simulink model "CVS Model"  (R2021a)
settings: Solver=VariableStepAuto  StartTime=0.0  StopTime=1.6  RelTol=1e-3
libraries: ee_lib x814, fl_lib x488, nesl_utility x60, simulink x4
(part 7 of 8)

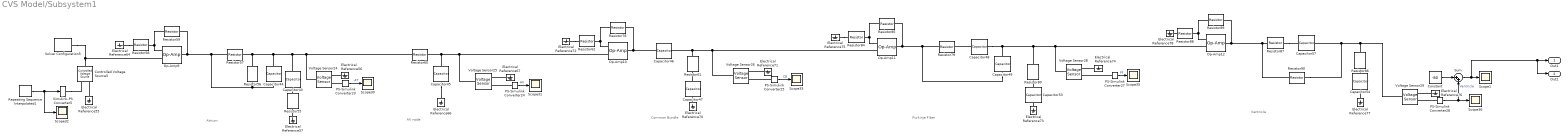
== system CVS Model/Subsystem1 ==
  note: Common Bundle
  note: Ventricle
  note: AV node
  note: Purkinje Fiber
  note: Atrium
  Capacitor43 : fl_lib/Electrical/Electrical Elements/Capacitor  c=80 uF  r=0 Ohm  g=0 1/Ohm  i_specify=off  i_priority=None  i=0 A  i_nominal_specify=off  i_nominal_unit=A  i_nominal_value=1  v_specify=off  v_priority=None  v=0 V  v_nominal_specify=off  v_nominal_unit=V  v_nominal_value=1  vc_specify=off  vc_priority=High  vc=0 V  vc_nominal_specify=off  vc_nominal_unit=V  vc_nominal_value=1
  Capacitor44 : fl_lib/Electrical/Electrical Elements/Capacitor  c=80 uF  r=0 Ohm  g=0 1/Ohm  i_specify=off  i_priority=None  i=0 A  i_nominal_specify=off  i_nominal_unit=A  i_nominal_value=1  v_specify=off  v_priority=None  v=0 V  v_nominal_specify=off  v_nominal_unit=V  v_nominal_value=1  vc_specify=off  vc_priority=High  vc=0 V  vc_nominal_specify=off  vc_nominal_unit=V  vc_nominal_value=1
  Capacitor45 : fl_lib/Electrical/Electrical Elements/Capacitor  c=20 uF  r=0 Ohm  g=0 1/Ohm  i_specify=off  i_priority=None  i=0 A  i_nominal_specify=off  i_nominal_unit=A  i_nominal_value=1  v_specify=off  v_priority=None  v=0 V  v_nominal_specify=off  v_nominal_unit=V  v_nominal_value=1  vc_specify=off  vc_priority=High  vc=0 V  vc_nominal_specify=off  vc_nominal_unit=V  vc_nominal_value=1
  Capacitor46 : fl_lib/Electrical/Electrical Elements/Capacitor  c=10 uF  r=1e-6 Ohm  g=0 1/Ohm  i_specify=off  i_priority=None  i=0 A  i_nominal_specify=off  i_nominal_unit=A  i_nominal_value=1  v_specify=off  v_priority=None  v=0 V  v_nominal_specify=off  v_nominal_unit=V  v_nominal_value=1  vc_specify=off  vc_priority=High  vc=0 V  vc_nominal_specify=off  vc_nominal_unit=V  vc_nominal_value=1
  Capacitor47 : fl_lib/Electrical/Electrical Elements/Capacitor  c=12 uF  r=0 Ohm  g=0 1/Ohm  i_specify=off  i_priority=None  i=0 A  i_nominal_specify=off  i_nominal_unit=A  i_nominal_value=1  v_specify=off  v_priority=None  v=0 V  v_nominal_specify=off  v_nominal_unit=V  v_nominal_value=1  vc_specify=off  vc_priority=High  vc=0 V  vc_nominal_specify=off  vc_nominal_unit=V  vc_nominal_value=1
  Capacitor48 : fl_lib/Electrical/Electrical Elements/Capacitor  c=20 uF  r=1e-6 Ohm  g=0 1/Ohm  i_specify=off  i_priority=None  i=0 A  i_nominal_specify=off  i_nominal_unit=A  i_nominal_value=1  v_specify=off  v_priority=None  v=0 V  v_nominal_specify=off  v_nominal_unit=V  v_nominal_value=1  vc_specify=off  vc_priority=High  vc=0 V  vc_nominal_specify=off  vc_nominal_unit=V  vc_nominal_value=1
  Capacitor49 : fl_lib/Electrical/Electrical Elements/Capacitor  c=30 uF  r=1e-6 Ohm  g=0 1/Ohm  i_specify=off  i_priority=None  i=0 A  i_nominal_specify=off  i_nominal_unit=A  i_nominal_value=1  v_specify=off  v_priority=None  v=0 V  v_nominal_specify=off  v_nominal_unit=V  v_nominal_value=1  vc_specify=off  vc_priority=High  vc=0 V  vc_nominal_specify=off  vc_nominal_unit=V  vc_nominal_value=1
  Capacitor53 : fl_lib/Electrical/Electrical Elements/Capacitor  c=50 uF  r=1e-6 Ohm  g=0 1/Ohm  i_specify=off  i_priority=None  i=0 A  i_nominal_specify=off  i_nominal_unit=A  i_nominal_value=1  v_specify=off  v_priority=None  v=0 V  v_nominal_specify=off  v_nominal_unit=V  v_nominal_value=1  vc_specify=off  vc_priority=High  vc=0 V  vc_nominal_specify=off  vc_nominal_unit=V  vc_nominal_value=1
  Capacitor54 : fl_lib/Electrical/Electrical Elements/Capacitor  c=2.5 uF  r=0 Ohm  g=0 1/Ohm  i_specify=off  i_priority=None  i=0 A  i_nominal_specify=off  i_nominal_unit=A  i_nominal_value=1  v_specify=off  v_priority=None  v=0 V  v_nominal_specify=off  v_nominal_unit=V  v_nominal_value=1  vc_specify=off  vc_priority=High  vc=0 V  vc_nominal_specify=off  vc_nominal_unit=V  vc_nominal_value=1
  Capacitor57 : fl_lib/Electrical/Electrical Elements/Capacitor  c=8 uF  r=0 Ohm  g=0 1/Ohm  i_specify=off  i_priority=None  i=0 A  i_nominal_specify=off  i_nominal_unit=A  i_nominal_value=1  v_specify=off  v_priority=None  v=0 V  v_nominal_specify=off  v_nominal_unit=V  v_nominal_value=1  vc_specify=off  vc_priority=High  vc=0 V  vc_nominal_specify=off  vc_nominal_unit=V  vc_nominal_value=1
  Constant : Constant  Value=-80
  Controlled Voltage Source5 : fl_lib/Electrical/Electrical Sources/Controlled Voltage Source
  Electrical Reference{55..57,64,66..67,70..78} (15 alike) : fl_lib/Electrical/Electrical Elements/Electrical Reference
  Op-Amp{9..12} (4 alike) : fl_lib/Electrical/Electrical Elements/Op-Amp  outI_specify=off  outI_priority=None  outI=0 A  outI_nominal_specify=off  outI_nominal_unit=A  outI_nominal_value=1
  PS-Simulink Converter{23..25,27..28} (5 alike) : nesl_utility/PS-Simulink Converter  PhysicalDomain=network_engine_domain  SubClassName=ps_output  LeftPortType=input  RightPortType=output  PseudoPeriodic=off  Frequencies=[]  Unit=inherit  AffineConversion=off
      settings: SourceProductBaseCode=PW,SS
  Repeating Sequence Interpolated1 : simulink/Sources/Repeating Sequence Interpolated  OutValues=[0 0.01 60 -3 0].'  TimeValues=[0 0.1 0.12 0.4 0.8].'  LookUpMeth=Interpolation-Use End Values  tsamp=0.0001  OutMin=[]  OutMax=[]  OutDataTypeStr=double  OutputDataTypeScalingMode=double  OutDataType=fixdt(0,8)  OutScaling=2^-10
  Resistor55 : fl_lib/Electrical/Electrical Elements/Resistor  R=0.4 kOhm  i_specify=off  i_priority=None  i=0 A  i_nominal_specify=off  i_nominal_unit=A  i_nominal_value=1  v_specify=off  v_priority=None  v=0 V  v_nominal_specify=off  v_nominal_unit=V  v_nominal_value=1
  Resistor56 : fl_lib/Electrical/Electrical Elements/Resistor  R=40 kOhm  i_specify=off  i_priority=None  i=0 A  i_nominal_specify=off  i_nominal_unit=A  i_nominal_value=1  v_specify=off  v_priority=None  v=0 V  v_nominal_specify=off  v_nominal_unit=V  v_nominal_value=1
  Resistor57 : fl_lib/Electrical/Electrical Elements/Resistor  R=0.3 kOhm  i_specify=off  i_priority=None  i=0 A  i_nominal_specify=off  i_nominal_unit=A  i_nominal_value=1  v_specify=off  v_priority=None  v=0 V  v_nominal_specify=off  v_nominal_unit=V  v_nominal_value=1
  Resistor58 : fl_lib/Electrical/Electrical Elements/Resistor  R=2 kOhm  i_specify=off  i_priority=None  i=0 A  i_nominal_specify=off  i_nominal_unit=A  i_nominal_value=1  v_specify=off  v_priority=None  v=0 V  v_nominal_specify=off  v_nominal_unit=V  v_nominal_value=1
  Resistor{59,78,85,89} (4 alike) : fl_lib/Electrical/Electrical Elements/Resistor  R=1.5 kOhm  i_specify=off  i_priority=None  i=0 A  i_nominal_specify=off  i_nominal_unit=A  i_nominal_value=1  v_specify=off  v_priority=None  v=0 V  v_nominal_specify=off  v_nominal_unit=V  v_nominal_value=1
  Resistor60 : fl_lib/Electrical/Electrical Elements/Resistor  R=0.4 kOhm  i_specify=off  i_priority=None  i=0 A  i_nominal_specify=off  i_nominal_unit=A  i_nominal_value=1  v_specify=off  v_priority=None  v=0 V  v_nominal_specify=off  v_nominal_unit=V  v_nominal_value=1
  Resistor61 : fl_lib/Electrical/Electrical Elements/Resistor  R=0.5 kOhm  i_specify=off  i_priority=None  i=0 A  i_nominal_specify=off  i_nominal_unit=A  i_nominal_value=1  v_specify=off  v_priority=None  v=0 V  v_nominal_specify=off  v_nominal_unit=V  v_nominal_value=1
  Resistor62 : fl_lib/Electrical/Electrical Elements/Resistor  R=2 kOhm  i_specify=off  i_priority=None  i=0 A  i_nominal_specify=off  i_nominal_unit=A  i_nominal_value=1  v_specify=off  v_priority=None  v=0 V  v_nominal_specify=off  v_nominal_unit=V  v_nominal_value=1
  Resistor79 : fl_lib/Electrical/Electrical Elements/Resistor  R=0.2 kOhm  i_specify=off  i_priority=None  i=0 A  i_nominal_specify=off  i_nominal_unit=A  i_nominal_value=1  v_specify=off  v_priority=None  v=0 V  v_nominal_specify=off  v_nominal_unit=V  v_nominal_value=1
  Resistor80 : fl_lib/Electrical/Electrical Elements/Resistor  R=0.4 kOhm  i_specify=off  i_priority=None  i=0 A  i_nominal_specify=off  i_nominal_unit=A  i_nominal_value=1  v_specify=off  v_priority=None  v=0 V  v_nominal_specify=off  v_nominal_unit=V  v_nominal_value=1
  Resistor84 : fl_lib/Electrical/Electrical Elements/Resistor  R=0.7 kOhm  i_specify=off  i_priority=None  i=0 A  i_nominal_specify=off  i_nominal_unit=A  i_nominal_value=1  v_specify=off  v_priority=None  v=0 V  v_nominal_specify=off  v_nominal_unit=V  v_nominal_value=1
  Resistor86 : fl_lib/Electrical/Electrical Elements/Resistor  R=1 kOhm  i_specify=off  i_priority=None  i=0 A  i_nominal_specify=off  i_nominal_unit=A  i_nominal_value=1  v_specify=off  v_priority=None  v=0 V  v_nominal_specify=off  v_nominal_unit=V  v_nominal_value=1
  Resistor87 : fl_lib/Electrical/Electrical Elements/Resistor  R=0.5 kOhm  i_specify=off  i_priority=None  i=0 A  i_nominal_specify=off  i_nominal_unit=A  i_nominal_value=1  v_specify=off  v_priority=None  v=0 V  v_nominal_specify=off  v_nominal_unit=V  v_nominal_value=1
  Resistor88 : fl_lib/Electrical/Electrical Elements/Resistor  R=3.5 kOhm  i_specify=off  i_priority=None  i=0 A  i_nominal_specify=off  i_nominal_unit=A  i_nominal_value=1  v_specify=off  v_priority=None  v=0 V  v_nominal_specify=off  v_nominal_unit=V  v_nominal_value=1
  Resistor90 : fl_lib/Electrical/Electrical Elements/Resistor  R=2.5 kOhm  i_specify=off  i_priority=None  i=0 A  i_nominal_specify=off  i_nominal_unit=A  i_nominal_value=1  v_specify=off  v_priority=None  v=0 V  v_nominal_specify=off  v_nominal_unit=V  v_nominal_value=1
  Scope{1,30..33,35..36} (7 alike) : Scope
  Simulink-PS Converter5 : nesl_utility/Simulink-PS Converter  PhysicalDomain=network_engine_domain  SubClassName=ps_input  LeftPortType=input  RightPortType=output  PseudoPeriodic=off  Frequencies=[]  NoiseDistribution=none  NoiseParameters=[]  Unit=1  AffineConversion=off  FilteringAndDerivatives=provide  SimscapeFilterOrder=1  InputFilterTimeConstant=0.001  UdotUserProvided=0
      settings: SourceProductBaseCode=PW,SS
  Solver Configuration5 : nesl_utility/Solver Configuration  PhysicalDomain=network_engine_domain  SubClassName=solver  LeftPortType=input  RightPortType=generic  Tones=[]  Harmonics=[]  SimulateNoise=off  Profile=off  UseLocalSampling=off  EnableSwitchedLinearOptims=on  FrequencyDomain=off  UseCCode=off  RelTol=0.001  AbsTol=1e-06  MinStep=1e-09  ToWorkspace=off  RevertToSquareIcSolve=off  NumHomotopyIterations=100  PhasorMode=off  PhasorModeNumHarmonics=1  DoDC=off  ResidualTolerance=1e-09  UseLocalSolver=off  LocalSolverChoice=NE_BACKWARD_EULER_ADVANCER  LocalSolverSampleTime=0.001  DoFixedCost=off  MaxNonlinIter=3  MaxModeIter=2  ComputeImpulses=off  ImpulseIterations=2  LinearAlgebra=auto  EquationFormulation=NE_TIME_EF  DelaysMemoryBudget=1024  AutomaticFiltering=on  FilteringTimeConstant=0.001  PartitionStorageMethod=AS_NEEDED  PartitionMemoryBudget=1024  PartitionMethod=ROBUST
      settings: SourceProductBaseCode=PW,SS
  Sum : Sum  Inputs=|++
  Voltage Sensor{24..26,28..29} (5 alike) : fl_lib/Electrical/Electrical Sensors/Voltage Sensor
  Out1 : Outport
  Out2 : Outport  Port=2
  wires:
  Repeating Sequence Interpolated1/1 -> Scope32/1, Simulink-PS Converter5/1
  PS-Simulink Converter24/1 -> Scope31/1  "AV"
  PS-Simulink Converter28/1 -> Sum/2, Scope36/1  "Ventricle"
  PS-Simulink Converter25/1 -> Scope33/1  "CB"
  PS-Simulink Converter23/1 -> Scope30/1  "AT"
  PS-Simulink Converter27/1 -> Scope35/1  "PF"
  Sum/1 -> Out2/1, Out1/1, Scope1/1
  Constant/1 -> Sum/1
  connections:
  PS-Simulink Converter24/LConn1 -- Voltage Sensor25/RConn1
  Resistor86/RConn1 -- Capacitor54/LConn1
  Resistor56/RConn1 -- Capacitor44/RConn1 -- Resistor57/LConn1 -- Resistor59/RConn1 -- Op-Amp9/RConn1
  Capacitor45/LConn1 -- Resistor60/RConn1 -- Op-Amp10/LConn2 -- Voltage Sensor25/LConn1
  Capacitor46/LConn1 -- Resistor78/RConn1 -- Op-Amp10/RConn1
  Electrical Reference55/LConn1 -- Controlled Voltage Source5/RConn2
  PS-Simulink Converter27/LConn1 -- Voltage Sensor28/RConn1
  Electrical Reference76/LConn1 -- Voltage Sensor29/RConn2
  Resistor85/RConn1 -- Op-Amp11/RConn1 -- Resistor79/LConn1 -- Capacitor49/RConn1
  Resistor89/RConn1 -- Op-Amp12/RConn1 -- Resistor87/LConn1 -- Resistor90/RConn1
  Electrical Reference78/LConn1 -- Resistor88/LConn1
  Resistor84/RConn1 -- Resistor85/LConn1 -- Op-Amp11/LConn1
  Resistor90/LConn1 -- Voltage Sensor29/LConn1 -- Resistor86/LConn1 -- Capacitor57/RConn1
  PS-Simulink Converter23/LConn1 -- Voltage Sensor24/RConn1
  Capacitor53/RConn1 -- Electrical Reference73/LConn1
  Capacitor47/RConn1 -- Electrical Reference70/LConn1
  Capacitor53/LConn1 -- Resistor80/RConn1
  PS-Simulink Converter28/LConn1 -- Voltage Sensor29/RConn1
  Controlled Voltage Source5/LConn1 -- Solver Configuration5/RConn1 -- Op-Amp9/LConn2
  Resistor62/RConn1 -- Resistor78/LConn1 -- Op-Amp10/LConn1
  Electrical Reference72/LConn1 -- Resistor62/LConn1
  Simulink-PS Converter5/RConn1 -- Controlled Voltage Source5/RConn1
  Electrical Reference64/LConn1 -- Resistor58/LConn1
  Capacitor45/RConn1 -- Electrical Reference66/LConn1
  PS-Simulink Converter25/LConn1 -- Voltage Sensor26/RConn1
  Electrical Reference75/LConn1 -- Resistor84/LConn1
  Capacitor48/LConn1 -- Resistor79/RConn1
  Electrical Reference74/LConn1 -- Voltage Sensor28/RConn2
  Electrical Reference71/LConn1 -- Voltage Sensor26/RConn2
  Resistor87/RConn1 -- Capacitor57/LConn1
  Electrical Reference67/LConn1 -- Voltage Sensor25/RConn2
  Electrical Reference77/LConn1 -- Capacitor54/RConn1
  Capacitor47/LConn1 -- Resistor61/RConn1
  Electrical Reference57/LConn1 -- Resistor55/RConn1
  Electrical Reference56/LConn1 -- Voltage Sensor24/RConn2
  Capacitor43/RConn1 -- Resistor55/LConn1
  Capacitor43/LConn1 -- Capacitor44/LConn1 -- Resistor56/LConn1 -- Resistor57/RConn1 -- Resistor60/LConn1 -- Voltage Sensor24/LConn1
  Resistor88/RConn1 -- Op-Amp12/LConn1 -- Resistor89/LConn1
  Resistor58/RConn1 -- Op-Amp9/LConn1 -- Resistor59/LConn1
  Voltage Sensor28/LConn1 -- Op-Amp12/LConn2 -- Resistor80/LConn1 -- Capacitor48/RConn1 -- Capacitor49/LConn1
  Capacitor46/RConn1 -- Resistor61/LConn1 -- Op-Amp11/LConn2 -- Voltage Sensor26/LConn1

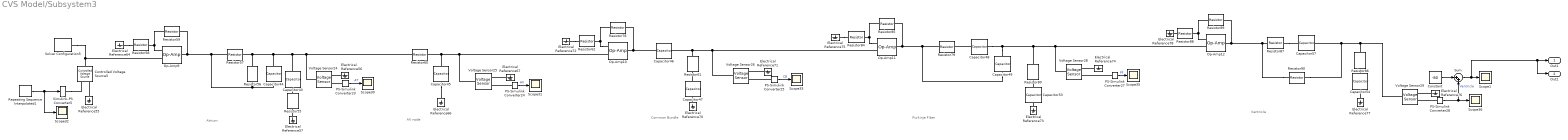
== system CVS Model/Subsystem3 ==
  note: Atrium
  note: Purkinje Fiber
  note: AV node
  note: Ventricle
  note: Common Bundle
  Capacitor43 : fl_lib/Electrical/Electrical Elements/Capacitor  c=80 uF  r=0 Ohm  g=0 1/Ohm  i_specify=off  i_priority=None  i=0 A  i_nominal_specify=off  i_nominal_unit=A  i_nominal_value=1  v_specify=off  v_priority=None  v=0 V  v_nominal_specify=off  v_nominal_unit=V  v_nominal_value=1  vc_specify=off  vc_priority=High  vc=0 V  vc_nominal_specify=off  vc_nominal_unit=V  vc_nominal_value=1
  Capacitor44 : fl_lib/Electrical/Electrical Elements/Capacitor  c=80 uF  r=0 Ohm  g=0 1/Ohm  i_specify=off  i_priority=None  i=0 A  i_nominal_specify=off  i_nominal_unit=A  i_nominal_value=1  v_specify=off  v_priority=None  v=0 V  v_nominal_specify=off  v_nominal_unit=V  v_nominal_value=1  vc_specify=off  vc_priority=High  vc=0 V  vc_nominal_specify=off  vc_nominal_unit=V  vc_nominal_value=1
  Capacitor45 : fl_lib/Electrical/Electrical Elements/Capacitor  c=20 uF  r=0 Ohm  g=0 1/Ohm  i_specify=off  i_priority=None  i=0 A  i_nominal_specify=off  i_nominal_unit=A  i_nominal_value=1  v_specify=off  v_priority=None  v=0 V  v_nominal_specify=off  v_nominal_unit=V  v_nominal_value=1  vc_specify=off  vc_priority=High  vc=0 V  vc_nominal_specify=off  vc_nominal_unit=V  vc_nominal_value=1
  Capacitor46 : fl_lib/Electrical/Electrical Elements/Capacitor  c=10 uF  r=1e-6 Ohm  g=0 1/Ohm  i_specify=off  i_priority=None  i=0 A  i_nominal_specify=off  i_nominal_unit=A  i_nominal_value=1  v_specify=off  v_priority=None  v=0 V  v_nominal_specify=off  v_nominal_unit=V  v_nominal_value=1  vc_specify=off  vc_priority=High  vc=0 V  vc_nominal_specify=off  vc_nominal_unit=V  vc_nominal_value=1
  Capacitor47 : fl_lib/Electrical/Electrical Elements/Capacitor  c=12 uF  r=0 Ohm  g=0 1/Ohm  i_specify=off  i_priority=None  i=0 A  i_nominal_specify=off  i_nominal_unit=A  i_nominal_value=1  v_specify=off  v_priority=None  v=0 V  v_nominal_specify=off  v_nominal_unit=V  v_nominal_value=1  vc_specify=off  vc_priority=High  vc=0 V  vc_nominal_specify=off  vc_nominal_unit=V  vc_nominal_value=1
  Capacitor48 : fl_lib/Electrical/Electrical Elements/Capacitor  c=20 uF  r=1e-6 Ohm  g=0 1/Ohm  i_specify=off  i_priority=None  i=0 A  i_nominal_specify=off  i_nominal_unit=A  i_nominal_value=1  v_specify=off  v_priority=None  v=0 V  v_nominal_specify=off  v_nominal_unit=V  v_nominal_value=1  vc_specify=off  vc_priority=High  vc=0 V  vc_nominal_specify=off  vc_nominal_unit=V  vc_nominal_value=1
  Capacitor49 : fl_lib/Electrical/Electrical Elements/Capacitor  c=30 uF  r=1e-6 Ohm  g=0 1/Ohm  i_specify=off  i_priority=None  i=0 A  i_nominal_specify=off  i_nominal_unit=A  i_nominal_value=1  v_specify=off  v_priority=None  v=0 V  v_nominal_specify=off  v_nominal_unit=V  v_nominal_value=1  vc_specify=off  vc_priority=High  vc=0 V  vc_nominal_specify=off  vc_nominal_unit=V  vc_nominal_value=1
  Capacitor53 : fl_lib/Electrical/Electrical Elements/Capacitor  c=50 uF  r=1e-6 Ohm  g=0 1/Ohm  i_specify=off  i_priority=None  i=0 A  i_nominal_specify=off  i_nominal_unit=A  i_nominal_value=1  v_specify=off  v_priority=None  v=0 V  v_nominal_specify=off  v_nominal_unit=V  v_nominal_value=1  vc_specify=off  vc_priority=High  vc=0 V  vc_nominal_specify=off  vc_nominal_unit=V  vc_nominal_value=1
  Capacitor54 : fl_lib/Electrical/Electrical Elements/Capacitor  c=2.5 uF  r=0 Ohm  g=0 1/Ohm  i_specify=off  i_priority=None  i=0 A  i_nominal_specify=off  i_nominal_unit=A  i_nominal_value=1  v_specify=off  v_priority=None  v=0 V  v_nominal_specify=off  v_nominal_unit=V  v_nominal_value=1  vc_specify=off  vc_priority=High  vc=0 V  vc_nominal_specify=off  vc_nominal_unit=V  vc_nominal_value=1
  Capacitor57 : fl_lib/Electrical/Electrical Elements/Capacitor  c=8 uF  r=0 Ohm  g=0 1/Ohm  i_specify=off  i_priority=None  i=0 A  i_nominal_specify=off  i_nominal_unit=A  i_nominal_value=1  v_specify=off  v_priority=None  v=0 V  v_nominal_specify=off  v_nominal_unit=V  v_nominal_value=1  vc_specify=off  vc_priority=High  vc=0 V  vc_nominal_specify=off  vc_nominal_unit=V  vc_nominal_value=1
  Constant : Constant  Value=-80
  Controlled Voltage Source5 : fl_lib/Electrical/Electrical Sources/Controlled Voltage Source
  Electrical Reference{55..57,64,66..67,70..78} (15 alike) : fl_lib/Electrical/Electrical Elements/Electrical Reference
  Op-Amp{9..12} (4 alike) : fl_lib/Electrical/Electrical Elements/Op-Amp  outI_specify=off  outI_priority=None  outI=0 A  outI_nominal_specify=off  outI_nominal_unit=A  outI_nominal_value=1
  PS-Simulink Converter{23..25,27..28} (5 alike) : nesl_utility/PS-Simulink Converter  PhysicalDomain=network_engine_domain  SubClassName=ps_output  LeftPortType=input  RightPortType=output  PseudoPeriodic=off  Frequencies=[]  Unit=inherit  AffineConversion=off
      settings: SourceProductBaseCode=PW,SS
  Repeating Sequence Interpolated1 : simulink/Sources/Repeating Sequence Interpolated  OutValues=[0 0.01 60 -3 0].'  TimeValues=[0 0.1 0.12 0.4 0.8].'  LookUpMeth=Interpolation-Use End Values  tsamp=0.0001  OutMin=[]  OutMax=[]  OutDataTypeStr=double  OutputDataTypeScalingMode=double  OutDataType=fixdt(0,8)  OutScaling=2^-10
  Resistor55 : fl_lib/Electrical/Electrical Elements/Resistor  R=0.4 kOhm  i_specify=off  i_priority=None  i=0 A  i_nominal_specify=off  i_nominal_unit=A  i_nominal_value=1  v_specify=off  v_priority=None  v=0 V  v_nominal_specify=off  v_nominal_unit=V  v_nominal_value=1
  Resistor56 : fl_lib/Electrical/Electrical Elements/Resistor  R=40 kOhm  i_specify=off  i_priority=None  i=0 A  i_nominal_specify=off  i_nominal_unit=A  i_nominal_value=1  v_specify=off  v_priority=None  v=0 V  v_nominal_specify=off  v_nominal_unit=V  v_nominal_value=1
  Resistor57 : fl_lib/Electrical/Electrical Elements/Resistor  R=0.3 kOhm  i_specify=off  i_priority=None  i=0 A  i_nominal_specify=off  i_nominal_unit=A  i_nominal_value=1  v_specify=off  v_priority=None  v=0 V  v_nominal_specify=off  v_nominal_unit=V  v_nominal_value=1
  Resistor58 : fl_lib/Electrical/Electrical Elements/Resistor  R=2 kOhm  i_specify=off  i_priority=None  i=0 A  i_nominal_specify=off  i_nominal_unit=A  i_nominal_value=1  v_specify=off  v_priority=None  v=0 V  v_nominal_specify=off  v_nominal_unit=V  v_nominal_value=1
  Resistor{59,78,85,89} (4 alike) : fl_lib/Electrical/Electrical Elements/Resistor  R=1.5 kOhm  i_specify=off  i_priority=None  i=0 A  i_nominal_specify=off  i_nominal_unit=A  i_nominal_value=1  v_specify=off  v_priority=None  v=0 V  v_nominal_specify=off  v_nominal_unit=V  v_nominal_value=1
  Resistor60 : fl_lib/Electrical/Electrical Elements/Resistor  R=0.4 kOhm  i_specify=off  i_priority=None  i=0 A  i_nominal_specify=off  i_nominal_unit=A  i_nominal_value=1  v_specify=off  v_priority=None  v=0 V  v_nominal_specify=off  v_nominal_unit=V  v_nominal_value=1
  Resistor61 : fl_lib/Electrical/Electrical Elements/Resistor  R=0.5 kOhm  i_specify=off  i_priority=None  i=0 A  i_nominal_specify=off  i_nominal_unit=A  i_nominal_value=1  v_specify=off  v_priority=None  v=0 V  v_nominal_specify=off  v_nominal_unit=V  v_nominal_value=1
  Resistor62 : fl_lib/Electrical/Electrical Elements/Resistor  R=2 kOhm  i_specify=off  i_priority=None  i=0 A  i_nominal_specify=off  i_nominal_unit=A  i_nominal_value=1  v_specify=off  v_priority=None  v=0 V  v_nominal_specify=off  v_nominal_unit=V  v_nominal_value=1
  Resistor79 : fl_lib/Electrical/Electrical Elements/Resistor  R=0.2 kOhm  i_specify=off  i_priority=None  i=0 A  i_nominal_specify=off  i_nominal_unit=A  i_nominal_value=1  v_specify=off  v_priority=None  v=0 V  v_nominal_specify=off  v_nominal_unit=V  v_nominal_value=1
  Resistor80 : fl_lib/Electrical/Electrical Elements/Resistor  R=0.4 kOhm  i_specify=off  i_priority=None  i=0 A  i_nominal_specify=off  i_nominal_unit=A  i_nominal_value=1  v_specify=off  v_priority=None  v=0 V  v_nominal_specify=off  v_nominal_unit=V  v_nominal_value=1
  Resistor84 : fl_lib/Electrical/Electrical Elements/Resistor  R=0.7 kOhm  i_specify=off  i_priority=None  i=0 A  i_nominal_specify=off  i_nominal_unit=A  i_nominal_value=1  v_specify=off  v_priority=None  v=0 V  v_nominal_specify=off  v_nominal_unit=V  v_nominal_value=1
  Resistor86 : fl_lib/Electrical/Electrical Elements/Resistor  R=1 kOhm  i_specify=off  i_priority=None  i=0 A  i_nominal_specify=off  i_nominal_unit=A  i_nominal_value=1  v_specify=off  v_priority=None  v=0 V  v_nominal_specify=off  v_nominal_unit=V  v_nominal_value=1
  Resistor87 : fl_lib/Electrical/Electrical Elements/Resistor  R=5 kOhm  i_specify=off  i_priority=None  i=0 A  i_nominal_specify=off  i_nominal_unit=A  i_nominal_value=1  v_specify=off  v_priority=None  v=0 V  v_nominal_specify=off  v_nominal_unit=V  v_nominal_value=1
  Resistor88 : fl_lib/Electrical/Electrical Elements/Resistor  R=3.5 kOhm  i_specify=off  i_priority=None  i=0 A  i_nominal_specify=off  i_nominal_unit=A  i_nominal_value=1  v_specify=off  v_priority=None  v=0 V  v_nominal_specify=off  v_nominal_unit=V  v_nominal_value=1
  Resistor90 : fl_lib/Electrical/Electrical Elements/Resistor  R=2.5 kOhm  i_specify=off  i_priority=None  i=0 A  i_nominal_specify=off  i_nominal_unit=A  i_nominal_value=1  v_specify=off  v_priority=None  v=0 V  v_nominal_specify=off  v_nominal_unit=V  v_nominal_value=1
  Scope{1,30..33,35..36} (7 alike) : Scope
  Simulink-PS Converter5 : nesl_utility/Simulink-PS Converter  PhysicalDomain=network_engine_domain  SubClassName=ps_input  LeftPortType=input  RightPortType=output  PseudoPeriodic=off  Frequencies=[]  NoiseDistribution=none  NoiseParameters=[]  Unit=1  AffineConversion=off  FilteringAndDerivatives=provide  SimscapeFilterOrder=1  InputFilterTimeConstant=0.001  UdotUserProvided=0
      settings: SourceProductBaseCode=PW,SS
  Solver Configuration5 : nesl_utility/Solver Configuration  PhysicalDomain=network_engine_domain  SubClassName=solver  LeftPortType=input  RightPortType=generic  Tones=[]  Harmonics=[]  SimulateNoise=off  Profile=off  UseLocalSampling=off  EnableSwitchedLinearOptims=on  FrequencyDomain=off  UseCCode=off  RelTol=0.001  AbsTol=1e-06  MinStep=1e-09  ToWorkspace=off  RevertToSquareIcSolve=off  NumHomotopyIterations=100  PhasorMode=off  PhasorModeNumHarmonics=1  DoDC=off  ResidualTolerance=1e-09  UseLocalSolver=off  LocalSolverChoice=NE_BACKWARD_EULER_ADVANCER  LocalSolverSampleTime=0.001  DoFixedCost=off  MaxNonlinIter=3  MaxModeIter=2  ComputeImpulses=off  ImpulseIterations=2  LinearAlgebra=auto  EquationFormulation=NE_TIME_EF  DelaysMemoryBudget=1024  AutomaticFiltering=on  FilteringTimeConstant=0.001  PartitionStorageMethod=AS_NEEDED  PartitionMemoryBudget=1024  PartitionMethod=ROBUST
      settings: SourceProductBaseCode=PW,SS
  Sum : Sum  Inputs=|++
  Voltage Sensor{24..26,28..29} (5 alike) : fl_lib/Electrical/Electrical Sensors/Voltage Sensor
  Out1 : Outport
  Out2 : Outport  Port=2
  wires:
  Constant/1 -> Sum/1
  Sum/1 -> Scope1/1, Out1/1, Out2/1
  PS-Simulink Converter27/1 -> Scope35/1  "PF"
  PS-Simulink Converter23/1 -> Scope30/1  "AT"
  PS-Simulink Converter25/1 -> Scope33/1  "CB"
  PS-Simulink Converter28/1 -> Scope36/1, Sum/2  "Ventricle"
  PS-Simulink Converter24/1 -> Scope31/1  "AV"
  Repeating Sequence Interpolated1/1 -> Simulink-PS Converter5/1, Scope32/1
  connections:
  Voltage Sensor26/LConn1 -- Op-Amp11/LConn2 -- Resistor61/LConn1 -- Capacitor46/RConn1
  Capacitor49/LConn1 -- Capacitor48/RConn1 -- Resistor80/LConn1 -- Op-Amp12/LConn2 -- Voltage Sensor28/LConn1
  Resistor59/LConn1 -- Op-Amp9/LConn1 -- Resistor58/RConn1
  Resistor89/LConn1 -- Op-Amp12/LConn1 -- Resistor88/RConn1
  Voltage Sensor24/LConn1 -- Resistor60/LConn1 -- Resistor57/RConn1 -- Resistor56/LConn1 -- Capacitor44/LConn1 -- Capacitor43/LConn1
  Capacitor43/RConn1 -- Resistor55/LConn1
  Electrical Reference56/LConn1 -- Voltage Sensor24/RConn2
  Electrical Reference57/LConn1 -- Resistor55/RConn1
  Capacitor47/LConn1 -- Resistor61/RConn1
  Electrical Reference77/LConn1 -- Capacitor54/RConn1
  Electrical Reference67/LConn1 -- Voltage Sensor25/RConn2
  Resistor87/RConn1 -- Capacitor57/LConn1
  Electrical Reference71/LConn1 -- Voltage Sensor26/RConn2
  Electrical Reference74/LConn1 -- Voltage Sensor28/RConn2
  Capacitor48/LConn1 -- Resistor79/RConn1
  Electrical Reference75/LConn1 -- Resistor84/LConn1
  PS-Simulink Converter25/LConn1 -- Voltage Sensor26/RConn1
  Capacitor45/RConn1 -- Electrical Reference66/LConn1
  Electrical Reference64/LConn1 -- Resistor58/LConn1
  Simulink-PS Converter5/RConn1 -- Controlled Voltage Source5/RConn1
  Electrical Reference72/LConn1 -- Resistor62/LConn1
  Op-Amp10/LConn1 -- Resistor78/LConn1 -- Resistor62/RConn1
  Op-Amp9/LConn2 -- Solver Configuration5/RConn1 -- Controlled Voltage Source5/LConn1
  PS-Simulink Converter28/LConn1 -- Voltage Sensor29/RConn1
  Capacitor53/LConn1 -- Resistor80/RConn1
  Capacitor47/RConn1 -- Electrical Reference70/LConn1
  Capacitor53/RConn1 -- Electrical Reference73/LConn1
  PS-Simulink Converter23/LConn1 -- Voltage Sensor24/RConn1
  Capacitor57/RConn1 -- Resistor86/LConn1 -- Voltage Sensor29/LConn1 -- Resistor90/LConn1
  Op-Amp11/LConn1 -- Resistor85/LConn1 -- Resistor84/RConn1
  Electrical Reference78/LConn1 -- Resistor88/LConn1
  Resistor90/RConn1 -- Resistor87/LConn1 -- Op-Amp12/RConn1 -- Resistor89/RConn1
  Capacitor49/RConn1 -- Resistor79/LConn1 -- Op-Amp11/RConn1 -- Resistor85/RConn1
  Electrical Reference76/LConn1 -- Voltage Sensor29/RConn2
  PS-Simulink Converter27/LConn1 -- Voltage Sensor28/RConn1
  Electrical Reference55/LConn1 -- Controlled Voltage Source5/RConn2
  Op-Amp10/RConn1 -- Resistor78/RConn1 -- Capacitor46/LConn1
  Voltage Sensor25/LConn1 -- Op-Amp10/LConn2 -- Resistor60/RConn1 -- Capacitor45/LConn1
  Op-Amp9/RConn1 -- Resistor59/RConn1 -- Resistor57/LConn1 -- Capacitor44/RConn1 -- Resistor56/RConn1
  Resistor86/RConn1 -- Capacitor54/LConn1
  PS-Simulink Converter24/LConn1 -- Voltage Sensor25/RConn1

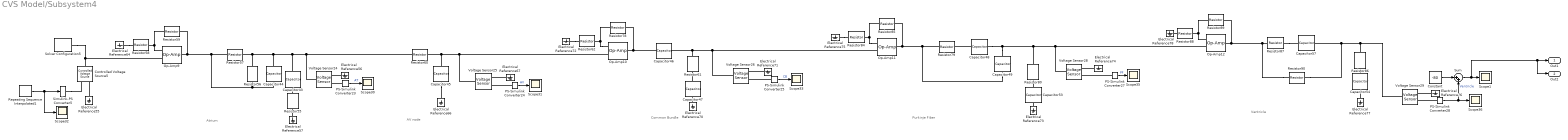
== system CVS Model/Subsystem4 ==
  note: Atrium
  note: Purkinje Fiber
  note: AV node
  note: Ventricle
  note: Common Bundle
  Capacitor43 : fl_lib/Electrical/Electrical Elements/Capacitor  c=80 uF  r=0 Ohm  g=0 1/Ohm  i_specify=off  i_priority=None  i=0 A  i_nominal_specify=off  i_nominal_unit=A  i_nominal_value=1  v_specify=off  v_priority=None  v=0 V  v_nominal_specify=off  v_nominal_unit=V  v_nominal_value=1  vc_specify=off  vc_priority=High  vc=0 V  vc_nominal_specify=off  vc_nominal_unit=V  vc_nominal_value=1
  Capacitor44 : fl_lib/Electrical/Electrical Elements/Capacitor  c=80 uF  r=0 Ohm  g=0 1/Ohm  i_specify=off  i_priority=None  i=0 A  i_nominal_specify=off  i_nominal_unit=A  i_nominal_value=1  v_specify=off  v_priority=None  v=0 V  v_nominal_specify=off  v_nominal_unit=V  v_nominal_value=1  vc_specify=off  vc_priority=High  vc=0 V  vc_nominal_specify=off  vc_nominal_unit=V  vc_nominal_value=1
  Capacitor45 : fl_lib/Electrical/Electrical Elements/Capacitor  c=20 uF  r=0 Ohm  g=0 1/Ohm  i_specify=off  i_priority=None  i=0 A  i_nominal_specify=off  i_nominal_unit=A  i_nominal_value=1  v_specify=off  v_priority=None  v=0 V  v_nominal_specify=off  v_nominal_unit=V  v_nominal_value=1  vc_specify=off  vc_priority=High  vc=0 V  vc_nominal_specify=off  vc_nominal_unit=V  vc_nominal_value=1
  Capacitor46 : fl_lib/Electrical/Electrical Elements/Capacitor  c=10 uF  r=1e-6 Ohm  g=0 1/Ohm  i_specify=off  i_priority=None  i=0 A  i_nominal_specify=off  i_nominal_unit=A  i_nominal_value=1  v_specify=off  v_priority=None  v=0 V  v_nominal_specify=off  v_nominal_unit=V  v_nominal_value=1  vc_specify=off  vc_priority=High  vc=0 V  vc_nominal_specify=off  vc_nominal_unit=V  vc_nominal_value=1
  Capacitor47 : fl_lib/Electrical/Electrical Elements/Capacitor  c=12 uF  r=0 Ohm  g=0 1/Ohm  i_specify=off  i_priority=None  i=0 A  i_nominal_specify=off  i_nominal_unit=A  i_nominal_value=1  v_specify=off  v_priority=None  v=0 V  v_nominal_specify=off  v_nominal_unit=V  v_nominal_value=1  vc_specify=off  vc_priority=High  vc=0 V  vc_nominal_specify=off  vc_nominal_unit=V  vc_nominal_value=1
  Capacitor48 : fl_lib/Electrical/Electrical Elements/Capacitor  c=20 uF  r=1e-6 Ohm  g=0 1/Ohm  i_specify=off  i_priority=None  i=0 A  i_nominal_specify=off  i_nominal_unit=A  i_nominal_value=1  v_specify=off  v_priority=None  v=0 V  v_nominal_specify=off  v_nominal_unit=V  v_nominal_value=1  vc_specify=off  vc_priority=High  vc=0 V  vc_nominal_specify=off  vc_nominal_unit=V  vc_nominal_value=1
  Capacitor49 : fl_lib/Electrical/Electrical Elements/Capacitor  c=30 uF  r=1e-6 Ohm  g=0 1/Ohm  i_specify=off  i_priority=None  i=0 A  i_nominal_specify=off  i_nominal_unit=A  i_nominal_value=1  v_specify=off  v_priority=None  v=0 V  v_nominal_specify=off  v_nominal_unit=V  v_nominal_value=1  vc_specify=off  vc_priority=High  vc=0 V  vc_nominal_specify=off  vc_nominal_unit=V  vc_nominal_value=1
  Capacitor53 : fl_lib/Electrical/Electrical Elements/Capacitor  c=50 uF  r=1e-6 Ohm  g=0 1/Ohm  i_specify=off  i_priority=None  i=0 A  i_nominal_specify=off  i_nominal_unit=A  i_nominal_value=1  v_specify=off  v_priority=None  v=0 V  v_nominal_specify=off  v_nominal_unit=V  v_nominal_value=1  vc_specify=off  vc_priority=High  vc=0 V  vc_nominal_specify=off  vc_nominal_unit=V  vc_nominal_value=1
  Capacitor54 : fl_lib/Electrical/Electrical Elements/Capacitor  c=2.5 uF  r=0 Ohm  g=0 1/Ohm  i_specify=off  i_priority=None  i=0 A  i_nominal_specify=off  i_nominal_unit=A  i_nominal_value=1  v_specify=off  v_priority=None  v=0 V  v_nominal_specify=off  v_nominal_unit=V  v_nominal_value=1  vc_specify=off  vc_priority=High  vc=0 V  vc_nominal_specify=off  vc_nominal_unit=V  vc_nominal_value=1
  Capacitor57 : fl_lib/Electrical/Electrical Elements/Capacitor  c=8 uF  r=0 Ohm  g=0 1/Ohm  i_specify=off  i_priority=None  i=0 A  i_nominal_specify=off  i_nominal_unit=A  i_nominal_value=1  v_specify=off  v_priority=None  v=0 V  v_nominal_specify=off  v_nominal_unit=V  v_nominal_value=1  vc_specify=off  vc_priority=High  vc=0 V  vc_nominal_specify=off  vc_nominal_unit=V  vc_nominal_value=1
  Constant : Constant  Value=-80
  Controlled Voltage Source5 : fl_lib/Electrical/Electrical Sources/Controlled Voltage Source
  Electrical Reference{55..57,64,66..67,70..78} (15 alike) : fl_lib/Electrical/Electrical Elements/Electrical Reference
  Op-Amp{9..12} (4 alike) : fl_lib/Electrical/Electrical Elements/Op-Amp  outI_specify=off  outI_priority=None  outI=0 A  outI_nominal_specify=off  outI_nominal_unit=A  outI_nominal_value=1
  PS-Simulink Converter{23..25,27..28} (5 alike) : nesl_utility/PS-Simulink Converter  PhysicalDomain=network_engine_domain  SubClassName=ps_output  LeftPortType=input  RightPortType=output  PseudoPeriodic=off  Frequencies=[]  Unit=inherit  AffineConversion=off
      settings: SourceProductBaseCode=PW,SS
  Repeating Sequence Interpolated1 : simulink/Sources/Repeating Sequence Interpolated  OutValues=[0 0.01 60 -3 0].'  TimeValues=[0 0.1 0.12 0.4 0.8].'  LookUpMeth=Interpolation-Use End Values  tsamp=0.0001  OutMin=[]  OutMax=[]  OutDataTypeStr=double  OutputDataTypeScalingMode=double  OutDataType=fixdt(0,8)  OutScaling=2^-10
  Resistor55 : fl_lib/Electrical/Electrical Elements/Resistor  R=0.4 kOhm  i_specify=off  i_priority=None  i=0 A  i_nominal_specify=off  i_nominal_unit=A  i_nominal_value=1  v_specify=off  v_priority=None  v=0 V  v_nominal_specify=off  v_nominal_unit=V  v_nominal_value=1
  Resistor56 : fl_lib/Electrical/Electrical Elements/Resistor  R=40 kOhm  i_specify=off  i_priority=None  i=0 A  i_nominal_specify=off  i_nominal_unit=A  i_nominal_value=1  v_specify=off  v_priority=None  v=0 V  v_nominal_specify=off  v_nominal_unit=V  v_nominal_value=1
  Resistor57 : fl_lib/Electrical/Electrical Elements/Resistor  R=0.3 kOhm  i_specify=off  i_priority=None  i=0 A  i_nominal_specify=off  i_nominal_unit=A  i_nominal_value=1  v_specify=off  v_priority=None  v=0 V  v_nominal_specify=off  v_nominal_unit=V  v_nominal_value=1
  Resistor58 : fl_lib/Electrical/Electrical Elements/Resistor  R=2 kOhm  i_specify=off  i_priority=None  i=0 A  i_nominal_specify=off  i_nominal_unit=A  i_nominal_value=1  v_specify=off  v_priority=None  v=0 V  v_nominal_specify=off  v_nominal_unit=V  v_nominal_value=1
  Resistor{59,78,85,89} (4 alike) : fl_lib/Electrical/Electrical Elements/Resistor  R=1.5 kOhm  i_specify=off  i_priority=None  i=0 A  i_nominal_specify=off  i_nominal_unit=A  i_nominal_value=1  v_specify=off  v_priority=None  v=0 V  v_nominal_specify=off  v_nominal_unit=V  v_nominal_value=1
  Resistor60 : fl_lib/Electrical/Electrical Elements/Resistor  R=0.4 kOhm  i_specify=off  i_priority=None  i=0 A  i_nominal_specify=off  i_nominal_unit=A  i_nominal_value=1  v_specify=off  v_priority=None  v=0 V  v_nominal_specify=off  v_nominal_unit=V  v_nominal_value=1
  Resistor61 : fl_lib/Electrical/Electrical Elements/Resistor  R=0.5 kOhm  i_specify=off  i_priority=None  i=0 A  i_nominal_specify=off  i_nominal_unit=A  i_nominal_value=1  v_specify=off  v_priority=None  v=0 V  v_nominal_specify=off  v_nominal_unit=V  v_nominal_value=1
  Resistor62 : fl_lib/Electrical/Electrical Elements/Resistor  R=2 kOhm  i_specify=off  i_priority=None  i=0 A  i_nominal_specify=off  i_nominal_unit=A  i_nominal_value=1  v_specify=off  v_priority=None  v=0 V  v_nominal_specify=off  v_nominal_unit=V  v_nominal_value=1
  Resistor79 : fl_lib/Electrical/Electrical Elements/Resistor  R=0.2 kOhm  i_specify=off  i_priority=None  i=0 A  i_nominal_specify=off  i_nominal_unit=A  i_nominal_value=1  v_specify=off  v_priority=None  v=0 V  v_nominal_specify=off  v_nominal_unit=V  v_nominal_value=1
  Resistor80 : fl_lib/Electrical/Electrical Elements/Resistor  R=0.4 kOhm  i_specify=off  i_priority=None  i=0 A  i_nominal_specify=off  i_nominal_unit=A  i_nominal_value=1  v_specify=off  v_priority=None  v=0 V  v_nominal_specify=off  v_nominal_unit=V  v_nominal_value=1
  Resistor84 : fl_lib/Electrical/Electrical Elements/Resistor  R=0.7 kOhm  i_specify=off  i_priority=None  i=0 A  i_nominal_specify=off  i_nominal_unit=A  i_nominal_value=1  v_specify=off  v_priority=None  v=0 V  v_nominal_specify=off  v_nominal_unit=V  v_nominal_value=1
  Resistor86 : fl_lib/Electrical/Electrical Elements/Resistor  R=1 kOhm  i_specify=off  i_priority=None  i=0 A  i_nominal_specify=off  i_nominal_unit=A  i_nominal_value=1  v_specify=off  v_priority=None  v=0 V  v_nominal_specify=off  v_nominal_unit=V  v_nominal_value=1
  Resistor87 : fl_lib/Electrical/Electrical Elements/Resistor  R=0.5 kOhm  i_specify=off  i_priority=None  i=0 A  i_nominal_specify=off  i_nominal_unit=A  i_nominal_value=1  v_specify=off  v_priority=None  v=0 V  v_nominal_specify=off  v_nominal_unit=V  v_nominal_value=1
  Resistor88 : fl_lib/Electrical/Electrical Elements/Resistor  R=3.5 kOhm  i_specify=off  i_priority=None  i=0 A  i_nominal_specify=off  i_nominal_unit=A  i_nominal_value=1  v_specify=off  v_priority=None  v=0 V  v_nominal_specify=off  v_nominal_unit=V  v_nominal_value=1
  Resistor90 : fl_lib/Electrical/Electrical Elements/Resistor  R=2.5 kOhm  i_specify=off  i_priority=None  i=0 A  i_nominal_specify=off  i_nominal_unit=A  i_nominal_value=1  v_specify=off  v_priority=None  v=0 V  v_nominal_specify=off  v_nominal_unit=V  v_nominal_value=1
  Scope{1,30..33,35..36} (7 alike) : Scope
  Simulink-PS Converter5 : nesl_utility/Simulink-PS Converter  PhysicalDomain=network_engine_domain  SubClassName=ps_input  LeftPortType=input  RightPortType=output  PseudoPeriodic=off  Frequencies=[]  NoiseDistribution=none  NoiseParameters=[]  Unit=1  AffineConversion=off  FilteringAndDerivatives=provide  SimscapeFilterOrder=1  InputFilterTimeConstant=0.001  UdotUserProvided=0
      settings: SourceProductBaseCode=PW,SS
  Solver Configuration5 : nesl_utility/Solver Configuration  PhysicalDomain=network_engine_domain  SubClassName=solver  LeftPortType=input  RightPortType=generic  Tones=[]  Harmonics=[]  SimulateNoise=off  Profile=off  UseLocalSampling=off  EnableSwitchedLinearOptims=on  FrequencyDomain=off  UseCCode=off  RelTol=0.001  AbsTol=1e-06  MinStep=1e-09  ToWorkspace=off  RevertToSquareIcSolve=off  NumHomotopyIterations=100  PhasorMode=off  PhasorModeNumHarmonics=1  DoDC=off  ResidualTolerance=1e-09  UseLocalSolver=off  LocalSolverChoice=NE_BACKWARD_EULER_ADVANCER  LocalSolverSampleTime=0.001  DoFixedCost=off  MaxNonlinIter=3  MaxModeIter=2  ComputeImpulses=off  ImpulseIterations=2  LinearAlgebra=auto  EquationFormulation=NE_TIME_EF  DelaysMemoryBudget=1024  AutomaticFiltering=on  FilteringTimeConstant=0.001  PartitionStorageMethod=AS_NEEDED  PartitionMemoryBudget=1024  PartitionMethod=ROBUST
      settings: SourceProductBaseCode=PW,SS
  Sum : Sum  Inputs=|++
  Voltage Sensor{24..26,28..29} (5 alike) : fl_lib/Electrical/Electrical Sensors/Voltage Sensor
  Out1 : Outport
  Out2 : Outport  Port=2
  wires:
  Constant/1 -> Sum/1
  Sum/1 -> Scope1/1, Out1/1, Out2/1
  PS-Simulink Converter27/1 -> Scope35/1  "PF"
  PS-Simulink Converter23/1 -> Scope30/1  "AT"
  PS-Simulink Converter25/1 -> Scope33/1  "CB"
  PS-Simulink Converter28/1 -> Scope36/1, Sum/2  "Ventricle"
  PS-Simulink Converter24/1 -> Scope31/1  "AV"
  Repeating Sequence Interpolated1/1 -> Simulink-PS Converter5/1, Scope32/1
  connections:
  Voltage Sensor26/LConn1 -- Op-Amp11/LConn2 -- Resistor61/LConn1 -- Capacitor46/RConn1
  Capacitor49/LConn1 -- Capacitor48/RConn1 -- Resistor80/LConn1 -- Op-Amp12/LConn2 -- Voltage Sensor28/LConn1
  Resistor59/LConn1 -- Op-Amp9/LConn1 -- Resistor58/RConn1
  Resistor89/LConn1 -- Op-Amp12/LConn1 -- Resistor88/RConn1
  Voltage Sensor24/LConn1 -- Resistor60/LConn1 -- Resistor57/RConn1 -- Resistor56/LConn1 -- Capacitor44/LConn1 -- Capacitor43/LConn1
  Capacitor43/RConn1 -- Resistor55/LConn1
  Electrical Reference56/LConn1 -- Voltage Sensor24/RConn2
  Electrical Reference57/LConn1 -- Resistor55/RConn1
  Capacitor47/LConn1 -- Resistor61/RConn1
  Electrical Reference77/LConn1 -- Capacitor54/RConn1
  Electrical Reference67/LConn1 -- Voltage Sensor25/RConn2
  Resistor87/RConn1 -- Capacitor57/LConn1
  Electrical Reference71/LConn1 -- Voltage Sensor26/RConn2
  Electrical Reference74/LConn1 -- Voltage Sensor28/RConn2
  Capacitor48/LConn1 -- Resistor79/RConn1
  Electrical Reference75/LConn1 -- Resistor84/LConn1
  PS-Simulink Converter25/LConn1 -- Voltage Sensor26/RConn1
  Capacitor45/RConn1 -- Electrical Reference66/LConn1
  Electrical Reference64/LConn1 -- Resistor58/LConn1
  Simulink-PS Converter5/RConn1 -- Controlled Voltage Source5/RConn1
  Electrical Reference72/LConn1 -- Resistor62/LConn1
  Op-Amp10/LConn1 -- Resistor78/LConn1 -- Resistor62/RConn1
  Op-Amp9/LConn2 -- Solver Configuration5/RConn1 -- Controlled Voltage Source5/LConn1
  PS-Simulink Converter28/LConn1 -- Voltage Sensor29/RConn1
  Capacitor53/LConn1 -- Resistor80/RConn1
  Capacitor47/RConn1 -- Electrical Reference70/LConn1
  Capacitor53/RConn1 -- Electrical Reference73/LConn1
  PS-Simulink Converter23/LConn1 -- Voltage Sensor24/RConn1
  Capacitor57/RConn1 -- Resistor86/LConn1 -- Voltage Sensor29/LConn1 -- Resistor90/LConn1
  Op-Amp11/LConn1 -- Resistor85/LConn1 -- Resistor84/RConn1
  Electrical Reference78/LConn1 -- Resistor88/LConn1
  Resistor90/RConn1 -- Resistor87/LConn1 -- Op-Amp12/RConn1 -- Resistor89/RConn1
  Capacitor49/RConn1 -- Resistor79/LConn1 -- Op-Amp11/RConn1 -- Resistor85/RConn1
  Electrical Reference76/LConn1 -- Voltage Sensor29/RConn2
  PS-Simulink Converter27/LConn1 -- Voltage Sensor28/RConn1
  Electrical Reference55/LConn1 -- Controlled Voltage Source5/RConn2
  Op-Amp10/RConn1 -- Resistor78/RConn1 -- Capacitor46/LConn1
  Voltage Sensor25/LConn1 -- Op-Amp10/LConn2 -- Resistor60/RConn1 -- Capacitor45/LConn1
  Op-Amp9/RConn1 -- Resistor59/RConn1 -- Resistor57/LConn1 -- Capacitor44/RConn1 -- Resistor56/RConn1
  Resistor86/RConn1 -- Capacitor54/LConn1
  PS-Simulink Converter24/LConn1 -- Voltage Sensor25/RConn1
